simulink model "MSFartoystyring_task2_5"  (R2019a)
settings: Solver=ode45  StartTime=tstart  StopTime=tstop  RelTol=1e-3  EnableMultiTasking=on
values from neighbouring files (symbols this model uses):
  c = 1    [run.m]    (also in run_task_2.m; run_task_2_chi_feedback.m; run_task_2_psi_feedback.m)
  Kd = -53    [run.m]    (also in run_task_2.m; run_task_2_chi_feedback.m; run_task_2_psi_feedback.m = -100)
  Ki = -1.6e-3    (= -0.0016)    [run.m]    (also in run_task_2.m; run_task_2_chi_feedback.m; run_task_2_psi_feedback.m = -2e-05)
  Ki_u = 1e-2    (= 0.01)    [run.m]    (also in run_task_2.m; run_task_2_chi_feedback.m; run_task_2_psi_feedback.m)
  Kp = -8    [run.m]    (also in run_task_2.m; run_task_2_chi_feedback.m; run_task_2_psi_feedback.m = -1)
  Kp_u = 50    [run.m]    (also in run_task_2.m; run_task_2_chi_feedback.m; run_task_2_psi_feedback.m)
  p0 = zeros(2,1)    [run.m]    (also in run_task_2.m; run_task_2_chi_feedback.m = zeros(1000, 700); run_task_2_psi_feedback.m = zeros(1000, 700))
  psi0 = 0    [run.m]    (also in run_task_2.m; run_task_2_chi_feedback.m = deg2rad(60); run_task_2_psi_feedback.m = deg2rad(60))
  r0 = 0    [run.m]    (also in run_task_2.m; run_task_2_chi_feedback.m; run_task_2_psi_feedback.m)
  tsamp = 10    [run.m]    (also in run_task_2.m; run_task_2_chi_feedback.m; run_task_2_psi_feedback.m)
  v0 = [3 0]'    [run.m]    (also in run_task_2.m; run_task_2_chi_feedback.m = [6 63]'; run_task_2_psi_feedback.m = [6 63]')
undefined symbols (not defined in the file or in its folder): msfartoystyring, WP
settings Model: ExtModeAutoUpdateStatusClock=off  Creator=christh  LastModifiedBy=magnusknaedal
settings DataIOCC: LimitDataPoints=on  SaveFormat=Array  ReturnWorkspaceOutputs=off
settings OptimizationCC: ExpressionDepthLimit=2147483647  InitFltsAndDblsToZero=on  LifeSpan=inf
settings DebuggingCC: UnderspecifiedInitializationDetection=Classic  MergeDetectMultiDrivingBlocksExec=none  SolverPrmCheckMsg=warning  FcnCallInpInsideContextMsg=warning  StateNameClashWarn=warning  SFUnexpectedBacktrackingDiag=warning  SFNoUnconditionalDefaultTransitionDiag=warning  SFExecutionAtInitializationDiag=none  ArithmeticOperatorsInVariantConditions=warning
settings HardwareCC: ProdBitPerPointer=32  ProdBitPerSizeT=32  ProdBitPerPtrDiffT=32  ProdLargestAtomicFloat=None  ProdIntDivRoundTo=Undefined  ProdEndianess=Unspecified  ProdWordSize=32  ProdHWDeviceType=32-bit Generic
settings ModelReferenceCC: PropagateSignalLabelsOutOfModel=off
settings SFSimCC: SimUseLocalCustomCode=off
settings RTWCC: RTWUseLocalCustomCode=off
settings CodeAppCC: StateflowObjectComments=on
settings GRTTargetCC: TargetLangStandard=C89/C90 (ANSI)  GeneratePreprocessorConditionals=Disable all  CombineOutputUpdateFcns=off  GRTInterface=on
settings ConfigComp: CovMetricSettings=dw  CovHtmlReporting=on  CovSaveCumulativeToWorkspaceVar=on  CovSaveSingleToWorkspaceVar=on  CovExternalEMLEnable=off

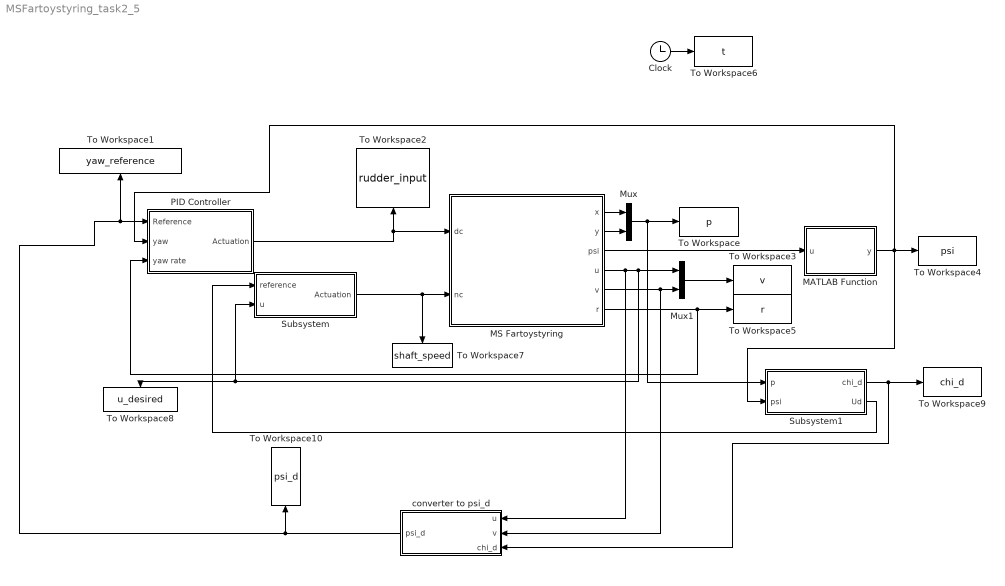
== system MSFartoystyring_task2_5 ==
  Clock : Clock
  MATLAB Function : MATLAB Function  TreatAsAtomicUnit=on
  MS Fartoystyring : Subsystem  mask(MS Fartoystyring for Assignment 3 G&C){x0=p0(1), y0=p0(2), u0=v0(1), v0=v0(2), psi0=psi0, r0=r0, c=c}
      mask prompts: x0 "x(t0) (m)"; y0 "y(t0) (m)"; u0 "u(t0) (m/s)"; v0 "v(t0) (m/s)"; psi0 "psi(t0) (rad)"; r0 "r(t0) (rad/s)"; c "current (0 or 1)"
      mask help:
      | Block corresponding to Figure 1 in the assignment text. Gives the response of the ship.
      |
      | The design speed of MS Fartoystyring is u=8.23 m/s.
      |
      | Input:
      | dc: commanded rudder (rad), dmax=25*pi/180
      | nc: commanded shaft speed (rad/s), nmax=85*2*pi/60
      |
      | Output:
      | x: north pos (m)
      | y: east pos (m)
      | u: surge (m/s)
      | v: sway (m/s)
      | psi: heading (rad)
      | r: yaw (rad/s)
      mask Help: Comments, bugs and help requests can be directed to the TA. Email on course website.
  Mux : Mux  Inputs=2
  Mux1 : Mux  Inputs=2
  PID Controller : Subsystem
  Subsystem : Subsystem
  Subsystem1 : Subsystem
  To Workspace : ToWorkspace  VariableName=p  SampleTime=tsamp
  To Workspace1 : ToWorkspace  VariableName=yaw_reference  SampleTime=tsamp
  To Workspace10 : ToWorkspace  VariableName=psi_d  SampleTime=tsamp
  To Workspace2 : ToWorkspace  VariableName=rudder_input  SampleTime=tsamp
  To Workspace3 : ToWorkspace  VariableName=v  SampleTime=tsamp
  To Workspace4 : ToWorkspace  VariableName=psi  SampleTime=tsamp
  To Workspace5 : ToWorkspace  VariableName=r  SampleTime=tsamp
  To Workspace6 : ToWorkspace  VariableName=t  SampleTime=tsamp
  To Workspace7 : ToWorkspace  VariableName=shaft_speed  SampleTime=tsamp
  To Workspace8 : ToWorkspace  VariableName=u_desired  SampleTime=tsamp
  To Workspace9 : ToWorkspace  VariableName=chi_d  SampleTime=tsamp
  converter to psi_d : Subsystem
  wires:
  Clock/1 -> To Workspace6/1
  MS Fartoystyring/1(x) -> Mux/1
  MS Fartoystyring/2(y) -> Mux/2
  MS Fartoystyring/4(u) -> Subsystem/2("u "), To Workspace8/1, Mux1/1, converter to psi_d/1(u)
  MS Fartoystyring/5(v) -> Mux1/2, converter to psi_d/2(v)
  Mux/1 -> Subsystem1/1(p), To Workspace/1
  Mux1/1 -> To Workspace3/1
  MS Fartoystyring/3(psi) -> MATLAB Function/1(u)
  MS Fartoystyring/6(r) -> PID Controller/3("yaw rate "), To Workspace5/1
  Subsystem/1("Actuation ") -> MS Fartoystyring/2(nc), To Workspace7/1
  PID Controller/1("Actuation ") -> To Workspace2/1, MS Fartoystyring/1(dc)
  Subsystem1/1(chi_d) -> converter to psi_d/3(chi_d), To Workspace9/1
  Subsystem1/2(Ud) -> Subsystem/1("reference ")
  MATLAB Function/1(y) -> Subsystem1/2(psi), PID Controller/2("yaw "), To Workspace4/1
  converter to psi_d/1(psi_d) -> To Workspace10/1, PID Controller/1(Reference), To Workspace1/1

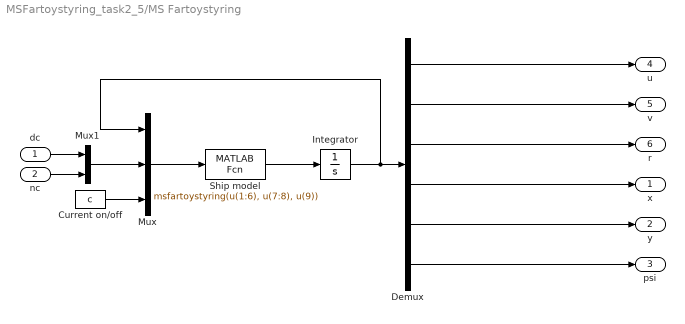
== system MSFartoystyring_task2_5/MS Fartoystyring ==
  dc : Inport
  nc : Inport  Port=2
  Current on/off : Constant  Value=c
  Demux : Demux  Outputs=6
  Integrator : Integrator  InitialCondition=[u0 v0 r0 x0 y0 psi0]'
  Mux : Mux  Inputs=3
  Mux1 : Mux  Inputs=2
  Ship model : MATLABFcn  MATLABFcn=msfartoystyring(u(1:6), u(7:8), u(9))  OutputDimensions=6
  x : Outport
  y : Outport  Port=2
  psi : Outport  Port=3
  u : Outport  Port=4
  v : Outport  Port=5
  r : Outport  Port=6
  wires:
  Integrator/1 -> Mux/1, Demux/1
  Mux1/1 -> Mux/2
  dc/1 -> Mux1/1
  nc/1 -> Mux1/2
  Current on/off/1 -> Mux/3
  Ship model/1 -> Integrator/1
  Mux/1 -> Ship model/1
  Demux/1 -> u/1
  Demux/2 -> v/1
  Demux/3 -> r/1
  Demux/4 -> x/1
  Demux/5 -> y/1
  Demux/6 -> psi/1

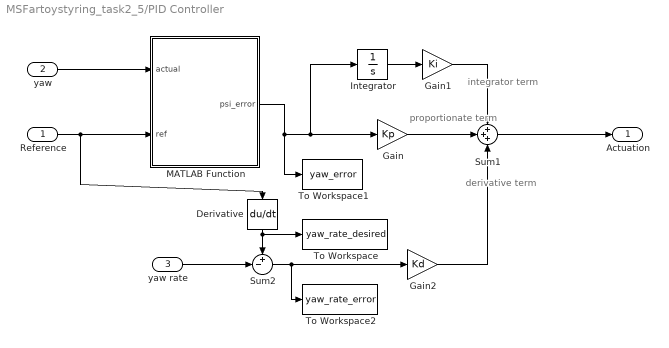
== system MSFartoystyring_task2_5/PID Controller ==
  note: derivative
      | term
  note: proportionate term
  note: integrator
      | term
  Reference : Inport
  "yaw " : Inport  Port=2
  "yaw rate " : Inport  Port=3
  Derivative : Derivative
  Gain : Gain  Gain=Kp
  Gain1 : Gain  Gain=Ki
  Gain2 : Gain  Gain=Kd
  Integrator : Integrator
  MATLAB Function : MATLAB Function  TreatAsAtomicUnit=on
  Sum1 : Sum  Inputs=+++
  Sum2 : Sum  Inputs=+-|
  To Workspace : ToWorkspace  VariableName=yaw_rate_desired  SampleTime=tsamp
  To Workspace1 : ToWorkspace  VariableName=yaw_error  SampleTime=tsamp
  To Workspace2 : ToWorkspace  VariableName=yaw_rate_error  SampleTime=tsamp
  "Actuation " : Outport
  wires:
  "yaw "/1 -> MATLAB Function/1(actual)
  Sum1/1 -> "Actuation "/1
  Gain/1 -> Sum1/2
  Derivative/1 -> To Workspace/1, Sum2/1
  "yaw rate "/1 -> Sum2/2
  Sum2/1 -> To Workspace2/1, Gain2/1
  Gain2/1 -> Sum1/3
  Gain1/1 -> Sum1/1
  Integrator/1 -> Gain1/1
  Reference/1 -> MATLAB Function/2(ref), Derivative/1
  MATLAB Function/1(psi_error) -> Gain/1, Integrator/1, To Workspace1/1

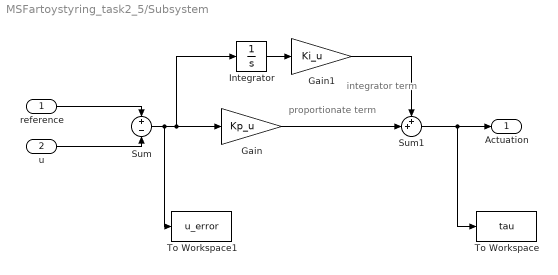
== system MSFartoystyring_task2_5/Subsystem ==
  note: proportionate term
  note: integrator
      | term
  "reference " : Inport
  "u " : Inport  Port=2
  Gain : Gain  Gain=Kp_u
  Gain1 : Gain  Gain=Ki_u
  Integrator : Integrator
  Sum : Sum  Inputs=+|-
  Sum1 : Sum  Inputs=++|
  To Workspace : ToWorkspace  VariableName=tau  SaveFormat=Timeseries  SampleTime=-1
  To Workspace1 : ToWorkspace  VariableName=u_error  SampleTime=tsamp
  "Actuation " : Outport
  wires:
  "reference "/1 -> Sum/1
  "u "/1 -> Sum/2
  Sum/1 -> To Workspace1/1, Integrator/1, Gain/1
  Sum1/1 -> To Workspace/1, "Actuation "/1
  Gain/1 -> Sum1/2
  Gain1/1 -> Sum1/1
  Integrator/1 -> Gain1/1

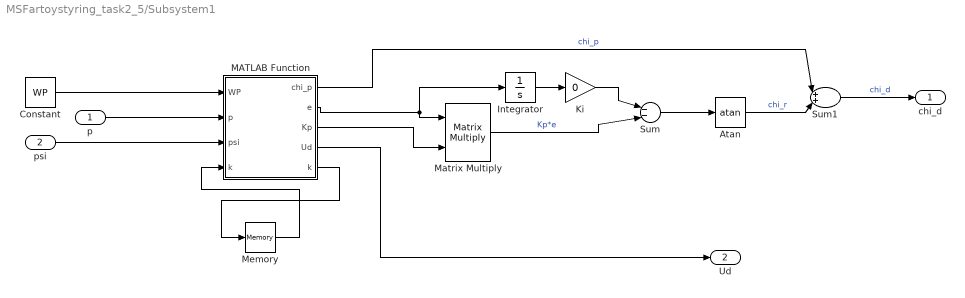
== system MSFartoystyring_task2_5/Subsystem1 ==
  p : Inport
  psi : Inport  Port=2
  Atan : Trigonometry  Operator=atan
  Constant : Constant  Value=WP
  Integrator : Integrator
  Ki : Gain  Gain=0
  MATLAB Function : MATLAB Function  TreatAsAtomicUnit=on  SystemSampleTime=tsamp
  Matrix Multiply : Product  Multiplication=Matrix(*)
  Memory : Memory  InitialCondition=1
  Sum : Sum  Inputs=|--|
  Sum1 : Sum  Inputs=|++|
  chi_d : Outport
  Ud : Outport  Port=2
  wires:
  p/1 -> MATLAB Function/2(p)
  psi/1 -> MATLAB Function/3(psi)
  Constant/1 -> MATLAB Function/1(WP)
  MATLAB Function/3(Kp) -> Matrix Multiply/2
  MATLAB Function/2(e) -> Matrix Multiply/1, Integrator/1
  Integrator/1 -> Ki/1
  Ki/1 -> Sum/1
  Matrix Multiply/1 -> Sum/2  "Kp*e"
  Sum/1 -> Atan/1
  Atan/1 -> Sum1/2  "chi_r"
  MATLAB Function/1(chi_p) -> Sum1/1  "chi_p"
  Sum1/1 -> chi_d/1  "chi_d"
  MATLAB Function/4(Ud) -> Ud/1
  MATLAB Function/5(k) -> Memory/1
  Memory/1 -> MATLAB Function/4("k ")

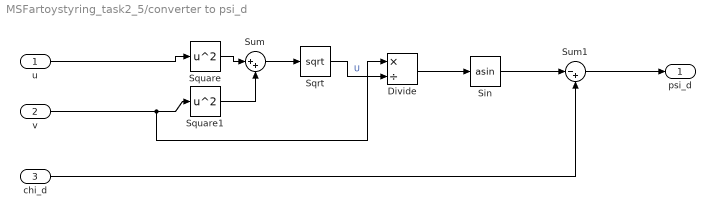
== system MSFartoystyring_task2_5/converter to psi_d ==
  u : Inport
  v : Inport  Port=2
  chi_d : Inport  Port=3
  Divide : Product  Inputs=*/
  Sin : Trigonometry  Operator=asin
  Sqrt : Sqrt  SaturateOnIntegerOverflow=on
  Square : Math  Operator=square  SaturateOnIntegerOverflow=on
  Square1 : Math  Operator=square  SaturateOnIntegerOverflow=on
  Sum : Sum  Inputs=|++
  Sum1 : Sum  Inputs=|-+
  psi_d : Outport
  wires:
  Square/1 -> Sum/1
  Square1/1 -> Sum/2
  Divide/1 -> Sin/1
  chi_d/1 -> Sum1/2
  Sum1/1 -> psi_d/1
  Sum/1 -> Sqrt/1
  u/1 -> Square/1
  v/1 -> Divide/1, Square1/1
  Sqrt/1 -> Divide/2  "U"
  Sin/1 -> Sum1/1

== matlab function MSFartoystyring_task2_5/PID Controller/MATLAB Function ==
  data: actual input; ref input; psi_error output
function psi_error = fcn(actual, ref)


psi_error = ssa(ref-actual,'rad');

== matlab function MSFartoystyring_task2_5/Subsystem1/MATLAB Function ==
  data: chi_p output; WP input; p input; e output; psi input; Kp output; Ud output; k output; k input
function [chi_p, e, Kp, Ud, k] = cte(WP, p, psi,k)

x = p(1); y = p(2);

R_tr = 1000;                         % turn radius
R_cos = 2.5*304.8;                    % radius for circle of acceptance = 2*Lpp

rad = (WP(1,k+1) - x)^2 + (WP(2,k+1)-y)^2; % squared distance to "next" waypoint
if rad <= R_cos^2 && k < length(WP)-1  
    k = k+1;                               % set current waypoint to next waypoint
end

alpha_k = atan2(WP(2, k+1)-WP(2, k), WP(1,k+1) - WP(1, k));
chi_p = alpha_k;                  

e = -(x - WP(1,k))*sin(alpha_k) + (y - WP(2,k))*cos(alpha_k); % cross track error

if (R_tr^2 - e^2) <= 0
    delta = 0.01;
else
    delta = sqrt(R_tr^2 - e^2);
end

Kp = 1/delta;         

Ud = 6.63;

if rad <= R_cos^2 && k == length(WP)
    Ud = 0;
end

end

== matlab function MSFartoystyring_task2_5/MATLAB Function ==
  data: u input; y output
function y = fcn(u)

y = ssa(u, 'rad');
